simulink model "Demo_PreScanCarSim3D_cs"  (Simulink 7.6)
settings: Solver=ode5  SolverMode=SingleTasking  StartTime=0.0  StopTime=68  FixedStep=1/400  RelTol=1e-3
PreLoadFcn:
  | check_NUTS_defined;
  | 
  | assignin('base',['model_closed_' bdroot],false);
InitFcn:
  | PreScanExperimentInitFcn(bdroot)
StopFcn:
  | PreScanExperimentStopFcn(bdroot)
undefined symbols (not defined in the file or in its folder): DiscIntNeverNeededParam, warningInitialVelocity, x0, x_ini_VRML, y_ini_VRML, z_ini_VRML
libraries: PreScanSimulinkLibrary x13, simulink_extras x5, PreScanUsefulBlocks x5, simulink x3, Solver_SF x1
(part 2 of 10)

== system Demo_PreScanCarSim3D_cs/GetSensors ==
  dummy : Inport
  GetSensors : M-S-Function  FunctionName=GetSensorsBlock  Parameters=TimeStep NrOfSensors
  tag scope: SimCoreSensors=global
  wires:
  GetSensors/1 -> [SimCoreSensors]
  dummy/1 -> GetSensors/1

== system Demo_PreScanCarSim3D_cs/HighwayOverhang_1 ==
  note: Resources
      |
      | 3: InformationSign\MatrixSign_Empty.png: MatrixSign Empty
      | 4: InformationSign\MatrixSign_End.png: MatrixSign End
      | 5: InformationSign\MatrixSign_GreenArrow.png: MatrixSign GreenArrow
      | 6: InformationSign\MatrixSign_RedCross.png: MatrixSign RedCross
      | 7: InformationSign\MatrixSign_Speed_50.png: MatrixSign Speed 50
      | 8: InformationSign\MatrixSign_Speed_70.png: MatrixSign Speed 70
      | 9: InformationSign\MatrixSign_Speed_90.png: MatrixSign Speed 90
      | 10: InformationSign\MatrixSign_Speed_120.png: MatrixSign Speed 120
      | 11: InformationSign\MatrixSign_Speed_130.png: MatrixSign Speed 130
      | 12: InformationSign\information.png: information
      | 13: InformationSign\TASS-international-logo.bmp: TASS-international-logo
  note: Resources
  Ground_{1..8} (8 alike) : Ground
  VISUMatrixSignLights_Mux : Subsystem  Tag=MuxMatrixSignLights
      settings: DeleteFcn=PreScanBlockDeleteFcn;
      mask Type: PreScan Mux Block:
  VISUMatrixSign_Mux : Subsystem  Tag=MuxMatrixSign
      settings: DeleteFcn=PreScanBlockDeleteFcn;
      mask Type: PreScan Mux Block:
  VISUMatrixSign_HighwayOverhang_1 : Outport  Tag=VisuMatrixSignOutport  SampleTime=20/400
  VISUMatrixSignLights_HighwayOverhang_1 : Outport  Tag=VisuMatrixSignLightsOutport  Port=2  SampleTime=20/400
  wires:
  Ground_8/1 -> VISUMatrixSign_Mux/4(MatrixSign_4)
  Ground_7/1 -> VISUMatrixSign_Mux/3(MatrixSign_3)
  Ground_6/1 -> VISUMatrixSign_Mux/2(MatrixSign_2)
  Ground_5/1 -> VISUMatrixSign_Mux/1(MatrixSign_1)
  Ground_4/1 -> VISUMatrixSignLights_Mux/4(MatrixSign_4)
  Ground_3/1 -> VISUMatrixSignLights_Mux/3(MatrixSign_3)
  Ground_2/1 -> VISUMatrixSignLights_Mux/2(MatrixSign_2)
  Ground_1/1 -> VISUMatrixSignLights_Mux/1(MatrixSign_1)
  VISUMatrixSignLights_Mux/1(MatrixSignLights) -> VISUMatrixSignLights_HighwayOverhang_1/1
  VISUMatrixSign_Mux/1(MatrixSigns) -> VISUMatrixSign_HighwayOverhang_1/1

== system Demo_PreScanCarSim3D_cs/HighwayOverhang_2 ==
  note: Resources
      |
      | 3: InformationSign\MatrixSign_Empty.png: MatrixSign Empty
      | 4: InformationSign\MatrixSign_End.png: MatrixSign End
      | 5: InformationSign\MatrixSign_GreenArrow.png: MatrixSign GreenArrow
      | 6: InformationSign\MatrixSign_RedCross.png: MatrixSign RedCross
      | 7: InformationSign\MatrixSign_Speed_50.png: MatrixSign Speed 50
      | 8: InformationSign\MatrixSign_Speed_70.png: MatrixSign Speed 70
      | 9: InformationSign\MatrixSign_Speed_90.png: MatrixSign Speed 90
      | 10: InformationSign\MatrixSign_Speed_120.png: MatrixSign Speed 120
      | 11: InformationSign\MatrixSign_Speed_130.png: MatrixSign Speed 130
      | 12: InformationSign\information.png: information
      | 13: InformationSign\TASS-international-logo.bmp: TASS-international-logo
  note: Resources
  Ground_{1..6} (6 alike) : Ground
  VISUMatrixSignLights_Mux : Subsystem  Tag=MuxMatrixSignLights
      settings: DeleteFcn=PreScanBlockDeleteFcn;
      mask Type: PreScan Mux Block:
  VISUMatrixSign_Mux : Subsystem  Tag=MuxMatrixSign
      settings: DeleteFcn=PreScanBlockDeleteFcn;
      mask Type: PreScan Mux Block:
  VISUMatrixSign_HighwayOverhang_2 : Outport  Tag=VisuMatrixSignOutport  SampleTime=20/400
  VISUMatrixSignLights_HighwayOverhang_2 : Outport  Tag=VisuMatrixSignLightsOutport  Port=2  SampleTime=20/400
  wires:
  Ground_6/1 -> VISUMatrixSign_Mux/3(MatrixSign_7)
  Ground_5/1 -> VISUMatrixSign_Mux/2(MatrixSign_6)
  Ground_4/1 -> VISUMatrixSign_Mux/1(MatrixSign_5)
  Ground_3/1 -> VISUMatrixSignLights_Mux/3(MatrixSign_7)
  Ground_2/1 -> VISUMatrixSignLights_Mux/2(MatrixSign_6)
  Ground_1/1 -> VISUMatrixSignLights_Mux/1(MatrixSign_5)
  VISUMatrixSignLights_Mux/1(MatrixSignLights) -> VISUMatrixSignLights_HighwayOverhang_2/1
  VISUMatrixSign_Mux/1(MatrixSigns) -> VISUMatrixSign_HighwayOverhang_2/1

== system Demo_PreScanCarSim3D_cs/HighwayOverhang_3 ==
  note: Resources
      |
      | 3: InformationSign\MatrixSign_Empty.png: MatrixSign Empty
      | 4: InformationSign\MatrixSign_End.png: MatrixSign End
      | 5: InformationSign\MatrixSign_GreenArrow.png: MatrixSign GreenArrow
      | 6: InformationSign\MatrixSign_RedCross.png: MatrixSign RedCross
      | 7: InformationSign\MatrixSign_Speed_50.png: MatrixSign Speed 50
      | 8: InformationSign\MatrixSign_Speed_70.png: MatrixSign Speed 70
      | 9: InformationSign\MatrixSign_Speed_90.png: MatrixSign Speed 90
      | 10: InformationSign\MatrixSign_Speed_120.png: MatrixSign Speed 120
      | 11: InformationSign\MatrixSign_Speed_130.png: MatrixSign Speed 130
      | 12: InformationSign\information.png: information
      | 13: InformationSign\TASS-international-logo.bmp: TASS-international-logo
  note: Resources
  Ground_{1..6} (6 alike) : Ground
  VISUMatrixSignLights_Mux : Subsystem  Tag=MuxMatrixSignLights
      settings: DeleteFcn=PreScanBlockDeleteFcn;
      mask Type: PreScan Mux Block:
  VISUMatrixSign_Mux : Subsystem  Tag=MuxMatrixSign
      settings: DeleteFcn=PreScanBlockDeleteFcn;
      mask Type: PreScan Mux Block:
  VISUMatrixSign_HighwayOverhang_3 : Outport  Tag=VisuMatrixSignOutport  SampleTime=20/400
  VISUMatrixSignLights_HighwayOverhang_3 : Outport  Tag=VisuMatrixSignLightsOutport  Port=2  SampleTime=20/400
  wires:
  Ground_6/1 -> VISUMatrixSign_Mux/3(MatrixSign_12)
  Ground_5/1 -> VISUMatrixSign_Mux/2(MatrixSign_11)
  Ground_4/1 -> VISUMatrixSign_Mux/1(MatrixSign_10)
  Ground_3/1 -> VISUMatrixSignLights_Mux/3(MatrixSign_12)
  Ground_2/1 -> VISUMatrixSignLights_Mux/2(MatrixSign_11)
  Ground_1/1 -> VISUMatrixSignLights_Mux/1(MatrixSign_10)
  VISUMatrixSignLights_Mux/1(MatrixSignLights) -> VISUMatrixSignLights_HighwayOverhang_3/1
  VISUMatrixSign_Mux/1(MatrixSigns) -> VISUMatrixSign_HighwayOverhang_3/1

== system Demo_PreScanCarSim3D_cs/HighwayOverhang_5 ==
  note: Resources
      |
      | 3: InformationSign\MatrixSign_Empty.png: MatrixSign Empty
      | 4: InformationSign\MatrixSign_End.png: MatrixSign End
      | 5: InformationSign\MatrixSign_GreenArrow.png: MatrixSign GreenArrow
      | 6: InformationSign\MatrixSign_RedCross.png: MatrixSign RedCross
      | 7: InformationSign\MatrixSign_Speed_50.png: MatrixSign Speed 50
      | 8: InformationSign\MatrixSign_Speed_70.png: MatrixSign Speed 70
      | 9: InformationSign\MatrixSign_Speed_90.png: MatrixSign Speed 90
      | 10: InformationSign\MatrixSign_Speed_120.png: MatrixSign Speed 120
      | 11: InformationSign\MatrixSign_Speed_130.png: MatrixSign Speed 130
      | 12: InformationSign\information.png: information
      | 13: InformationSign\TASS-international-logo.bmp: TASS-international-logo
  note: Resources
  Ground_{1..6} (6 alike) : Ground
  VISUMatrixSignLights_Mux : Subsystem  Tag=MuxMatrixSignLights
      settings: DeleteFcn=PreScanBlockDeleteFcn;
      mask Type: PreScan Mux Block:
  VISUMatrixSign_Mux : Subsystem  Tag=MuxMatrixSign
      settings: DeleteFcn=PreScanBlockDeleteFcn;
      mask Type: PreScan Mux Block:
  VISUMatrixSign_HighwayOverhang_5 : Outport  Tag=VisuMatrixSignOutport  SampleTime=20/400
  VISUMatrixSignLights_HighwayOverhang_5 : Outport  Tag=VisuMatrixSignLightsOutport  Port=2  SampleTime=20/400
  wires:
  Ground_6/1 -> VISUMatrixSign_Mux/3(MatrixSign_20)
  Ground_5/1 -> VISUMatrixSign_Mux/2(MatrixSign_19)
  Ground_4/1 -> VISUMatrixSign_Mux/1(MatrixSign_18)
  Ground_3/1 -> VISUMatrixSignLights_Mux/3(MatrixSign_20)
  Ground_2/1 -> VISUMatrixSignLights_Mux/2(MatrixSign_19)
  Ground_1/1 -> VISUMatrixSignLights_Mux/1(MatrixSign_18)
  VISUMatrixSignLights_Mux/1(MatrixSignLights) -> VISUMatrixSignLights_HighwayOverhang_5/1
  VISUMatrixSign_Mux/1(MatrixSigns) -> VISUMatrixSign_HighwayOverhang_5/1

== system Demo_PreScanCarSim3D_cs/Lightpost_1 ==

== system Demo_PreScanCarSim3D_cs/Lightpost_10 ==

== system Demo_PreScanCarSim3D_cs/Lightpost_11 ==

== system Demo_PreScanCarSim3D_cs/Lightpost_12 ==

== system Demo_PreScanCarSim3D_cs/Lightpost_13 ==

== system Demo_PreScanCarSim3D_cs/Lightpost_14 ==

== system Demo_PreScanCarSim3D_cs/Lightpost_15 ==

== system Demo_PreScanCarSim3D_cs/Lightpost_16 ==

== system Demo_PreScanCarSim3D_cs/Lightpost_17 ==

== system Demo_PreScanCarSim3D_cs/Lightpost_18 ==

== system Demo_PreScanCarSim3D_cs/Lightpost_19 ==

== system Demo_PreScanCarSim3D_cs/Lightpost_2 ==

== system Demo_PreScanCarSim3D_cs/Lightpost_20 ==

== system Demo_PreScanCarSim3D_cs/Lightpost_21 ==

== system Demo_PreScanCarSim3D_cs/Lightpost_22 ==

== system Demo_PreScanCarSim3D_cs/Lightpost_23 ==

== system Demo_PreScanCarSim3D_cs/Lightpost_24 ==

== system Demo_PreScanCarSim3D_cs/Lightpost_25 ==

== system Demo_PreScanCarSim3D_cs/Lightpost_26 ==

== system Demo_PreScanCarSim3D_cs/Lightpost_27 ==

== system Demo_PreScanCarSim3D_cs/Lightpost_28 ==

== system Demo_PreScanCarSim3D_cs/Lightpost_29 ==

== system Demo_PreScanCarSim3D_cs/Lightpost_30 ==

== system Demo_PreScanCarSim3D_cs/Lightpost_31 ==

== system Demo_PreScanCarSim3D_cs/Lightpost_32 ==

== system Demo_PreScanCarSim3D_cs/Lightpost_33 ==

== system Demo_PreScanCarSim3D_cs/Lightpost_34 ==

== system Demo_PreScanCarSim3D_cs/Lightpost_35 ==

== system Demo_PreScanCarSim3D_cs/Lightpost_36 ==

== system Demo_PreScanCarSim3D_cs/Lightpost_7 ==

== system Demo_PreScanCarSim3D_cs/Lightpost_8 ==

== system Demo_PreScanCarSim3D_cs/Lightpost_9 ==

== system Demo_PreScanCarSim3D_cs/SELF_Audi_A8_1 ==
  Selector : Selector  IndexMode=Zero-based  IndexOptions=Starting index (dialog)  Indices=PortIndex  OutputSizes=PortWidth(1)
  U : Outport
  wires:
  Selector/1 -> U/1
  [SimCoreSensors] -> Selector/1

== system Demo_PreScanCarSim3D_cs/SELF_Box_1 ==
  Selector : Selector  IndexMode=Zero-based  IndexOptions=Starting index (dialog)  Indices=PortIndex  OutputSizes=PortWidth(1)
  U : Outport
  wires:
  Selector/1 -> U/1
  [SimCoreSensors] -> Selector/1

== system Demo_PreScanCarSim3D_cs/SELF_Box_2 ==
  Selector : Selector  IndexMode=Zero-based  IndexOptions=Starting index (dialog)  Indices=PortIndex  OutputSizes=PortWidth(1)
  U : Outport
  wires:
  Selector/1 -> U/1
  [SimCoreSensors] -> Selector/1

== system Demo_PreScanCarSim3D_cs/SELF_Box_3 ==
  Selector : Selector  IndexMode=Zero-based  IndexOptions=Starting index (dialog)  Indices=PortIndex  OutputSizes=PortWidth(1)
  U : Outport
  wires:
  Selector/1 -> U/1
  [SimCoreSensors] -> Selector/1

== system Demo_PreScanCarSim3D_cs/SELF_Box_4 ==
  Selector : Selector  IndexMode=Zero-based  IndexOptions=Starting index (dialog)  Indices=PortIndex  OutputSizes=PortWidth(1)
  U : Outport
  wires:
  Selector/1 -> U/1
  [SimCoreSensors] -> Selector/1

== system Demo_PreScanCarSim3D_cs/STATE_Audi_A8_1 ==
  State : Inport  SampleTime=TimeStep
  Acceleration : Subsystem  mask(ToSensorWorld){PortName=Acceleration_Audi_A8_1, PortIndex=66, PortWidth=3, TimeStep=20/400}
      mask prompts: PortName "Port Name [-]"; PortIndex "Index [-]"; PortWidth "Port Dimensions [-]"; TimeStep "Upload Period [s]"
      mask help: Sends signal(s) from Simulink to the Sensor World
      mask Help:
      | Sends signal(s) from Simulink to the Sensor World.
      | 
      | - Port Name [-]: specifies the name of the output terminal of the Simulink block.
      | - Index [-]: specifies the start position in the output vector sent to the Sensor World
      | - Port dimensions [-]: specifies the width (number of scalars) of the output port
      | - Upload period [s]: specifies the upload period (in seconds) of the port.
      mask Display: port_label('input', 1, PortName)
  Demux : Demux  Outputs=5
  Position : Subsystem  mask(ToSensorWorld){PortName=Position_Audi_A8_1, PortIndex=60, PortWidth=3, TimeStep=20/400}
      mask prompts: PortName "Port Name [-]"; PortIndex "Index [-]"; PortWidth "Port Dimensions [-]"; TimeStep "Upload Period [s]"
      mask help: Sends signal(s) from Simulink to the Sensor World
      mask Help:
      | Sends signal(s) from Simulink to the Sensor World.
      | 
      | - Port Name [-]: specifies the name of the output terminal of the Simulink block.
      | - Index [-]: specifies the start position in the output vector sent to the Sensor World
      | - Port dimensions [-]: specifies the width (number of scalars) of the output port
      | - Upload period [s]: specifies the upload period (in seconds) of the port.
      mask Display: port_label('input', 1, PortName)
  RPY : Subsystem  mask(ToSensorWorld){PortName=RPY_Audi_A8_1, PortIndex=69, PortWidth=3, TimeStep=20/400}
      mask prompts: PortName "Port Name [-]"; PortIndex "Index [-]"; PortWidth "Port Dimensions [-]"; TimeStep "Upload Period [s]"
      mask help: Sends signal(s) from Simulink to the Sensor World
      mask Help:
      | Sends signal(s) from Simulink to the Sensor World.
      | 
      | - Port Name [-]: specifies the name of the output terminal of the Simulink block.
      | - Index [-]: specifies the start position in the output vector sent to the Sensor World
      | - Port dimensions [-]: specifies the width (number of scalars) of the output port
      | - Upload period [s]: specifies the upload period (in seconds) of the port.
      mask Display: port_label('input', 1, PortName)
  Velocity : Subsystem  mask(ToSensorWorld){PortName=Velocity_Audi_A8_1, PortIndex=63, PortWidth=3, TimeStep=20/400}
      mask prompts: PortName "Port Name [-]"; PortIndex "Index [-]"; PortWidth "Port Dimensions [-]"; TimeStep "Upload Period [s]"
      mask help: Sends signal(s) from Simulink to the Sensor World
      mask Help:
      | Sends signal(s) from Simulink to the Sensor World.
      | 
      | - Port Name [-]: specifies the name of the output terminal of the Simulink block.
      | - Index [-]: specifies the start position in the output vector sent to the Sensor World
      | - Port dimensions [-]: specifies the width (number of scalars) of the output port
      | - Upload period [s]: specifies the upload period (in seconds) of the port.
      mask Display: port_label('input', 1, PortName)
  iniBODYAngles wrtVEH [rad] : Constant  Value=[Roll0 Pitch0 0]  SampleTime=TimeStep
  iniVEHAngles wrtGLOB [rad] : Constant  Value=[0 0 Yaw0]  SampleTime=TimeStep
  iniVEHposition wrtGLOB [m] : Constant  Value=[x0 y0 z0]  SampleTime=TimeStep
  state2FullState : PreScanSimulinkLibrary/state2FullState  SystemSampleTime=-1
  velRPY : Subsystem  mask(ToSensorWorld){PortName=velRPY_Audi_A8_1, PortIndex=72, PortWidth=3, TimeStep=20/400}
      mask prompts: PortName "Port Name [-]"; PortIndex "Index [-]"; PortWidth "Port Dimensions [-]"; TimeStep "Upload Period [s]"
      mask help: Sends signal(s) from Simulink to the Sensor World
      mask Help:
      | Sends signal(s) from Simulink to the Sensor World.
      | 
      | - Port Name [-]: specifies the name of the output terminal of the Simulink block.
      | - Index [-]: specifies the start position in the output vector sent to the Sensor World
      | - Port dimensions [-]: specifies the width (number of scalars) of the output port
      | - Upload period [s]: specifies the upload period (in seconds) of the port.
      mask Display: port_label('input', 1, PortName)
  wires:
  Demux/5 -> velRPY/1(Y)
  Demux/4 -> RPY/1(Y)
  Demux/3 -> Acceleration/1(Y)
  Demux/2 -> Velocity/1(Y)
  Demux/1 -> Position/1(Y)
  State/1 -> state2FullState/1
  state2FullState/1 -> Demux/1
  iniVEHposition wrtGLOB [m]/1 -> state2FullState/2
  iniBODYAngles wrtVEH [rad]/1 -> state2FullState/3
  iniVEHAngles wrtGLOB [rad]/1 -> state2FullState/4

== system Demo_PreScanCarSim3D_cs/STATE_Box_1 ==
  State : Inport  SampleTime=TimeStep
  Acceleration : Subsystem  mask(ToSensorWorld){PortName=Acceleration_Box_1, PortIndex=6, PortWidth=3, TimeStep=20/400}
      mask prompts: PortName "Port Name [-]"; PortIndex "Index [-]"; PortWidth "Port Dimensions [-]"; TimeStep "Upload Period [s]"
      mask help: Sends signal(s) from Simulink to the Sensor World
      mask Help:
      | Sends signal(s) from Simulink to the Sensor World.
      | 
      | - Port Name [-]: specifies the name of the output terminal of the Simulink block.
      | - Index [-]: specifies the start position in the output vector sent to the Sensor World
      | - Port dimensions [-]: specifies the width (number of scalars) of the output port
      | - Upload period [s]: specifies the upload period (in seconds) of the port.
      mask Display: port_label('input', 1, PortName)
  Demux : Demux  Outputs=5
  Position : Subsystem  mask(ToSensorWorld){PortName=Position_Box_1, PortIndex=0, PortWidth=3, TimeStep=20/400}
      mask prompts: PortName "Port Name [-]"; PortIndex "Index [-]"; PortWidth "Port Dimensions [-]"; TimeStep "Upload Period [s]"
      mask help: Sends signal(s) from Simulink to the Sensor World
      mask Help:
      | Sends signal(s) from Simulink to the Sensor World.
      | 
      | - Port Name [-]: specifies the name of the output terminal of the Simulink block.
      | - Index [-]: specifies the start position in the output vector sent to the Sensor World
      | - Port dimensions [-]: specifies the width (number of scalars) of the output port
      | - Upload period [s]: specifies the upload period (in seconds) of the port.
      mask Display: port_label('input', 1, PortName)
  RPY : Subsystem  mask(ToSensorWorld){PortName=RPY_Box_1, PortIndex=9, PortWidth=3, TimeStep=20/400}
      mask prompts: PortName "Port Name [-]"; PortIndex "Index [-]"; PortWidth "Port Dimensions [-]"; TimeStep "Upload Period [s]"
      mask help: Sends signal(s) from Simulink to the Sensor World
      mask Help:
      | Sends signal(s) from Simulink to the Sensor World.
      | 
      | - Port Name [-]: specifies the name of the output terminal of the Simulink block.
      | - Index [-]: specifies the start position in the output vector sent to the Sensor World
      | - Port dimensions [-]: specifies the width (number of scalars) of the output port
      | - Upload period [s]: specifies the upload period (in seconds) of the port.
      mask Display: port_label('input', 1, PortName)
  Velocity : Subsystem  mask(ToSensorWorld){PortName=Velocity_Box_1, PortIndex=3, PortWidth=3, TimeStep=20/400}
      mask prompts: PortName "Port Name [-]"; PortIndex "Index [-]"; PortWidth "Port Dimensions [-]"; TimeStep "Upload Period [s]"
      mask help: Sends signal(s) from Simulink to the Sensor World
      mask Help:
      | Sends signal(s) from Simulink to the Sensor World.
      | 
      | - Port Name [-]: specifies the name of the output terminal of the Simulink block.
      | - Index [-]: specifies the start position in the output vector sent to the Sensor World
      | - Port dimensions [-]: specifies the width (number of scalars) of the output port
      | - Upload period [s]: specifies the upload period (in seconds) of the port.
      mask Display: port_label('input', 1, PortName)
  iniBODYAngles wrtVEH [rad] : Constant  Value=[Roll0 Pitch0 0]  SampleTime=TimeStep
  iniVEHAngles wrtGLOB [rad] : Constant  Value=[0 0 Yaw0]  SampleTime=TimeStep
  iniVEHposition wrtGLOB [m] : Constant  Value=[x0 y0 z0]  SampleTime=TimeStep
  state2FullState : PreScanSimulinkLibrary/state2FullState  SystemSampleTime=-1
  velRPY : Subsystem  mask(ToSensorWorld){PortName=velRPY_Box_1, PortIndex=12, PortWidth=3, TimeStep=20/400}
      mask prompts: PortName "Port Name [-]"; PortIndex "Index [-]"; PortWidth "Port Dimensions [-]"; TimeStep "Upload Period [s]"
      mask help: Sends signal(s) from Simulink to the Sensor World
      mask Help:
      | Sends signal(s) from Simulink to the Sensor World.
      | 
      | - Port Name [-]: specifies the name of the output terminal of the Simulink block.
      | - Index [-]: specifies the start position in the output vector sent to the Sensor World
      | - Port dimensions [-]: specifies the width (number of scalars) of the output port
      | - Upload period [s]: specifies the upload period (in seconds) of the port.
      mask Display: port_label('input', 1, PortName)
  wires:
  Demux/5 -> velRPY/1(Y)
  Demux/4 -> RPY/1(Y)
  Demux/3 -> Acceleration/1(Y)
  Demux/2 -> Velocity/1(Y)
  Demux/1 -> Position/1(Y)
  State/1 -> state2FullState/1
  state2FullState/1 -> Demux/1
  iniVEHposition wrtGLOB [m]/1 -> state2FullState/2
  iniBODYAngles wrtVEH [rad]/1 -> state2FullState/3
  iniVEHAngles wrtGLOB [rad]/1 -> state2FullState/4

== system Demo_PreScanCarSim3D_cs/STATE_Box_2 ==
  State : Inport  SampleTime=TimeStep
  Acceleration : Subsystem  mask(ToSensorWorld){PortName=Acceleration_Box_2, PortIndex=21, PortWidth=3, TimeStep=20/400}
      mask prompts: PortName "Port Name [-]"; PortIndex "Index [-]"; PortWidth "Port Dimensions [-]"; TimeStep "Upload Period [s]"
      mask help: Sends signal(s) from Simulink to the Sensor World
      mask Help:
      | Sends signal(s) from Simulink to the Sensor World.
      | 
      | - Port Name [-]: specifies the name of the output terminal of the Simulink block.
      | - Index [-]: specifies the start position in the output vector sent to the Sensor World
      | - Port dimensions [-]: specifies the width (number of scalars) of the output port
      | - Upload period [s]: specifies the upload period (in seconds) of the port.
      mask Display: port_label('input', 1, PortName)
  Demux : Demux  Outputs=5
  Position : Subsystem  mask(ToSensorWorld){PortName=Position_Box_2, PortIndex=15, PortWidth=3, TimeStep=20/400}
      mask prompts: PortName "Port Name [-]"; PortIndex "Index [-]"; PortWidth "Port Dimensions [-]"; TimeStep "Upload Period [s]"
      mask help: Sends signal(s) from Simulink to the Sensor World
      mask Help:
      | Sends signal(s) from Simulink to the Sensor World.
      | 
      | - Port Name [-]: specifies the name of the output terminal of the Simulink block.
      | - Index [-]: specifies the start position in the output vector sent to the Sensor World
      | - Port dimensions [-]: specifies the width (number of scalars) of the output port
      | - Upload period [s]: specifies the upload period (in seconds) of the port.
      mask Display: port_label('input', 1, PortName)
  RPY : Subsystem  mask(ToSensorWorld){PortName=RPY_Box_2, PortIndex=24, PortWidth=3, TimeStep=20/400}
      mask prompts: PortName "Port Name [-]"; PortIndex "Index [-]"; PortWidth "Port Dimensions [-]"; TimeStep "Upload Period [s]"
      mask help: Sends signal(s) from Simulink to the Sensor World
      mask Help:
      | Sends signal(s) from Simulink to the Sensor World.
      | 
      | - Port Name [-]: specifies the name of the output terminal of the Simulink block.
      | - Index [-]: specifies the start position in the output vector sent to the Sensor World
      | - Port dimensions [-]: specifies the width (number of scalars) of the output port
      | - Upload period [s]: specifies the upload period (in seconds) of the port.
      mask Display: port_label('input', 1, PortName)
  Velocity : Subsystem  mask(ToSensorWorld){PortName=Velocity_Box_2, PortIndex=18, PortWidth=3, TimeStep=20/400}
      mask prompts: PortName "Port Name [-]"; PortIndex "Index [-]"; PortWidth "Port Dimensions [-]"; TimeStep "Upload Period [s]"
      mask help: Sends signal(s) from Simulink to the Sensor World
      mask Help:
      | Sends signal(s) from Simulink to the Sensor World.
      | 
      | - Port Name [-]: specifies the name of the output terminal of the Simulink block.
      | - Index [-]: specifies the start position in the output vector sent to the Sensor World
      | - Port dimensions [-]: specifies the width (number of scalars) of the output port
      | - Upload period [s]: specifies the upload period (in seconds) of the port.
      mask Display: port_label('input', 1, PortName)
  iniBODYAngles wrtVEH [rad] : Constant  Value=[Roll0 Pitch0 0]  SampleTime=TimeStep
  iniVEHAngles wrtGLOB [rad] : Constant  Value=[0 0 Yaw0]  SampleTime=TimeStep
  iniVEHposition wrtGLOB [m] : Constant  Value=[x0 y0 z0]  SampleTime=TimeStep
  state2FullState : PreScanSimulinkLibrary/state2FullState  SystemSampleTime=-1
  velRPY : Subsystem  mask(ToSensorWorld){PortName=velRPY_Box_2, PortIndex=27, PortWidth=3, TimeStep=20/400}
      mask prompts: PortName "Port Name [-]"; PortIndex "Index [-]"; PortWidth "Port Dimensions [-]"; TimeStep "Upload Period [s]"
      mask help: Sends signal(s) from Simulink to the Sensor World
      mask Help:
      | Sends signal(s) from Simulink to the Sensor World.
      | 
      | - Port Name [-]: specifies the name of the output terminal of the Simulink block.
      | - Index [-]: specifies the start position in the output vector sent to the Sensor World
      | - Port dimensions [-]: specifies the width (number of scalars) of the output port
      | - Upload period [s]: specifies the upload period (in seconds) of the port.
      mask Display: port_label('input', 1, PortName)
  wires:
  Demux/5 -> velRPY/1(Y)
  Demux/4 -> RPY/1(Y)
  Demux/3 -> Acceleration/1(Y)
  Demux/2 -> Velocity/1(Y)
  Demux/1 -> Position/1(Y)
  State/1 -> state2FullState/1
  state2FullState/1 -> Demux/1
  iniVEHposition wrtGLOB [m]/1 -> state2FullState/2
  iniBODYAngles wrtVEH [rad]/1 -> state2FullState/3
  iniVEHAngles wrtGLOB [rad]/1 -> state2FullState/4

== system Demo_PreScanCarSim3D_cs/STATE_Box_3 ==
  State : Inport  SampleTime=TimeStep
  Acceleration : Subsystem  mask(ToSensorWorld){PortName=Acceleration_Box_3, PortIndex=36, PortWidth=3, TimeStep=20/400}
      mask prompts: PortName "Port Name [-]"; PortIndex "Index [-]"; PortWidth "Port Dimensions [-]"; TimeStep "Upload Period [s]"
      mask help: Sends signal(s) from Simulink to the Sensor World
      mask Help:
      | Sends signal(s) from Simulink to the Sensor World.
      | 
      | - Port Name [-]: specifies the name of the output terminal of the Simulink block.
      | - Index [-]: specifies the start position in the output vector sent to the Sensor World
      | - Port dimensions [-]: specifies the width (number of scalars) of the output port
      | - Upload period [s]: specifies the upload period (in seconds) of the port.
      mask Display: port_label('input', 1, PortName)
  Demux : Demux  Outputs=5
  Position : Subsystem  mask(ToSensorWorld){PortName=Position_Box_3, PortIndex=30, PortWidth=3, TimeStep=20/400}
      mask prompts: PortName "Port Name [-]"; PortIndex "Index [-]"; PortWidth "Port Dimensions [-]"; TimeStep "Upload Period [s]"
      mask help: Sends signal(s) from Simulink to the Sensor World
      mask Help:
      | Sends signal(s) from Simulink to the Sensor World.
      | 
      | - Port Name [-]: specifies the name of the output terminal of the Simulink block.
      | - Index [-]: specifies the start position in the output vector sent to the Sensor World
      | - Port dimensions [-]: specifies the width (number of scalars) of the output port
      | - Upload period [s]: specifies the upload period (in seconds) of the port.
      mask Display: port_label('input', 1, PortName)
  RPY : Subsystem  mask(ToSensorWorld){PortName=RPY_Box_3, PortIndex=39, PortWidth=3, TimeStep=20/400}
      mask prompts: PortName "Port Name [-]"; PortIndex "Index [-]"; PortWidth "Port Dimensions [-]"; TimeStep "Upload Period [s]"
      mask help: Sends signal(s) from Simulink to the Sensor World
      mask Help:
      | Sends signal(s) from Simulink to the Sensor World.
      | 
      | - Port Name [-]: specifies the name of the output terminal of the Simulink block.
      | - Index [-]: specifies the start position in the output vector sent to the Sensor World
      | - Port dimensions [-]: specifies the width (number of scalars) of the output port
      | - Upload period [s]: specifies the upload period (in seconds) of the port.
      mask Display: port_label('input', 1, PortName)
  Velocity : Subsystem  mask(ToSensorWorld){PortName=Velocity_Box_3, PortIndex=33, PortWidth=3, TimeStep=20/400}
      mask prompts: PortName "Port Name [-]"; PortIndex "Index [-]"; PortWidth "Port Dimensions [-]"; TimeStep "Upload Period [s]"
      mask help: Sends signal(s) from Simulink to the Sensor World
      mask Help:
      | Sends signal(s) from Simulink to the Sensor World.
      | 
      | - Port Name [-]: specifies the name of the output terminal of the Simulink block.
      | - Index [-]: specifies the start position in the output vector sent to the Sensor World
      | - Port dimensions [-]: specifies the width (number of scalars) of the output port
      | - Upload period [s]: specifies the upload period (in seconds) of the port.
      mask Display: port_label('input', 1, PortName)
  iniBODYAngles wrtVEH [rad] : Constant  Value=[Roll0 Pitch0 0]  SampleTime=TimeStep
  iniVEHAngles wrtGLOB [rad] : Constant  Value=[0 0 Yaw0]  SampleTime=TimeStep
  iniVEHposition wrtGLOB [m] : Constant  Value=[x0 y0 z0]  SampleTime=TimeStep
  state2FullState : PreScanSimulinkLibrary/state2FullState  SystemSampleTime=-1
  velRPY : Subsystem  mask(ToSensorWorld){PortName=velRPY_Box_3, PortIndex=42, PortWidth=3, TimeStep=20/400}
      mask prompts: PortName "Port Name [-]"; PortIndex "Index [-]"; PortWidth "Port Dimensions [-]"; TimeStep "Upload Period [s]"
      mask help: Sends signal(s) from Simulink to the Sensor World
      mask Help:
      | Sends signal(s) from Simulink to the Sensor World.
      | 
      | - Port Name [-]: specifies the name of the output terminal of the Simulink block.
      | - Index [-]: specifies the start position in the output vector sent to the Sensor World
      | - Port dimensions [-]: specifies the width (number of scalars) of the output port
      | - Upload period [s]: specifies the upload period (in seconds) of the port.
      mask Display: port_label('input', 1, PortName)
  wires:
  Demux/5 -> velRPY/1(Y)
  Demux/4 -> RPY/1(Y)
  Demux/3 -> Acceleration/1(Y)
  Demux/2 -> Velocity/1(Y)
  Demux/1 -> Position/1(Y)
  State/1 -> state2FullState/1
  state2FullState/1 -> Demux/1
  iniVEHposition wrtGLOB [m]/1 -> state2FullState/2
  iniBODYAngles wrtVEH [rad]/1 -> state2FullState/3
  iniVEHAngles wrtGLOB [rad]/1 -> state2FullState/4

== system Demo_PreScanCarSim3D_cs/STATE_Box_4 ==
  State : Inport  SampleTime=TimeStep
  Acceleration : Subsystem  mask(ToSensorWorld){PortName=Acceleration_Box_4, PortIndex=51, PortWidth=3, TimeStep=20/400}
      mask prompts: PortName "Port Name [-]"; PortIndex "Index [-]"; PortWidth "Port Dimensions [-]"; TimeStep "Upload Period [s]"
      mask help: Sends signal(s) from Simulink to the Sensor World
      mask Help:
      | Sends signal(s) from Simulink to the Sensor World.
      | 
      | - Port Name [-]: specifies the name of the output terminal of the Simulink block.
      | - Index [-]: specifies the start position in the output vector sent to the Sensor World
      | - Port dimensions [-]: specifies the width (number of scalars) of the output port
      | - Upload period [s]: specifies the upload period (in seconds) of the port.
      mask Display: port_label('input', 1, PortName)
  Demux : Demux  Outputs=5
  Position : Subsystem  mask(ToSensorWorld){PortName=Position_Box_4, PortIndex=45, PortWidth=3, TimeStep=20/400}
      mask prompts: PortName "Port Name [-]"; PortIndex "Index [-]"; PortWidth "Port Dimensions [-]"; TimeStep "Upload Period [s]"
      mask help: Sends signal(s) from Simulink to the Sensor World
      mask Help:
      | Sends signal(s) from Simulink to the Sensor World.
      | 
      | - Port Name [-]: specifies the name of the output terminal of the Simulink block.
      | - Index [-]: specifies the start position in the output vector sent to the Sensor World
      | - Port dimensions [-]: specifies the width (number of scalars) of the output port
      | - Upload period [s]: specifies the upload period (in seconds) of the port.
      mask Display: port_label('input', 1, PortName)
  RPY : Subsystem  mask(ToSensorWorld){PortName=RPY_Box_4, PortIndex=54, PortWidth=3, TimeStep=20/400}
      mask prompts: PortName "Port Name [-]"; PortIndex "Index [-]"; PortWidth "Port Dimensions [-]"; TimeStep "Upload Period [s]"
      mask help: Sends signal(s) from Simulink to the Sensor World
      mask Help:
      | Sends signal(s) from Simulink to the Sensor World.
      | 
      | - Port Name [-]: specifies the name of the output terminal of the Simulink block.
      | - Index [-]: specifies the start position in the output vector sent to the Sensor World
      | - Port dimensions [-]: specifies the width (number of scalars) of the output port
      | - Upload period [s]: specifies the upload period (in seconds) of the port.
      mask Display: port_label('input', 1, PortName)
  Velocity : Subsystem  mask(ToSensorWorld){PortName=Velocity_Box_4, PortIndex=48, PortWidth=3, TimeStep=20/400}
      mask prompts: PortName "Port Name [-]"; PortIndex "Index [-]"; PortWidth "Port Dimensions [-]"; TimeStep "Upload Period [s]"
      mask help: Sends signal(s) from Simulink to the Sensor World
      mask Help:
      | Sends signal(s) from Simulink to the Sensor World.
      | 
      | - Port Name [-]: specifies the name of the output terminal of the Simulink block.
      | - Index [-]: specifies the start position in the output vector sent to the Sensor World
      | - Port dimensions [-]: specifies the width (number of scalars) of the output port
      | - Upload period [s]: specifies the upload period (in seconds) of the port.
      mask Display: port_label('input', 1, PortName)
  iniBODYAngles wrtVEH [rad] : Constant  Value=[Roll0 Pitch0 0]  SampleTime=TimeStep
  iniVEHAngles wrtGLOB [rad] : Constant  Value=[0 0 Yaw0]  SampleTime=TimeStep
  iniVEHposition wrtGLOB [m] : Constant  Value=[x0 y0 z0]  SampleTime=TimeStep
  state2FullState : PreScanSimulinkLibrary/state2FullState  SystemSampleTime=-1
  velRPY : Subsystem  mask(ToSensorWorld){PortName=velRPY_Box_4, PortIndex=57, PortWidth=3, TimeStep=20/400}
      mask prompts: PortName "Port Name [-]"; PortIndex "Index [-]"; PortWidth "Port Dimensions [-]"; TimeStep "Upload Period [s]"
      mask help: Sends signal(s) from Simulink to the Sensor World
      mask Help:
      | Sends signal(s) from Simulink to the Sensor World.
      | 
      | - Port Name [-]: specifies the name of the output terminal of the Simulink block.
      | - Index [-]: specifies the start position in the output vector sent to the Sensor World
      | - Port dimensions [-]: specifies the width (number of scalars) of the output port
      | - Upload period [s]: specifies the upload period (in seconds) of the port.
      mask Display: port_label('input', 1, PortName)
  wires:
  Demux/5 -> velRPY/1(Y)
  Demux/4 -> RPY/1(Y)
  Demux/3 -> Acceleration/1(Y)
  Demux/2 -> Velocity/1(Y)
  Demux/1 -> Position/1(Y)
  State/1 -> state2FullState/1
  state2FullState/1 -> Demux/1
  iniVEHposition wrtGLOB [m]/1 -> state2FullState/2
  iniBODYAngles wrtVEH [rad]/1 -> state2FullState/3
  iniVEHAngles wrtGLOB [rad]/1 -> state2FullState/4

== system Demo_PreScanCarSim3D_cs/SetActuators ==
  Bus Creator : BusCreator  Inputs=1
  Data Store Read : DataStoreRead  DataStoreName=SimCoreActuators  SampleTime=TimeStep
  SendActuators : M-S-Function  FunctionName=SendActuatorsBlock  Parameters=TimeStep NrOfActuators
  dummy : Outport
  tag scope: SimCoreInfo=global
  wires:
  Bus Creator/1 -> [SimCoreInfo]  "SimCore"
  SendActuators/2 -> Bus Creator/1  "ComputationTime[s]"
  SendActuators/1 -> dummy/1
  Data Store Read/1 -> SendActuators/1

== system Demo_PreScanCarSim3D_cs/SimCoreInfo ==
  Bus Selector : BusSelector  OutputSignals=ComputationTime[s]
  Time : Scope
      settings: TimeRange=10  YMin=0  YMax=0.5  SaveName=ComputationTime
  wires:
  Bus Selector/1 -> Time/1  "<ComputationTime[s]>"
  [SimCoreInfo] -> Bus Selector/1

== system Demo_PreScanCarSim3D_cs/TrafficLightRoadSideNL_1 ==
  Ground_1 : Ground
  Ground_2 : Ground
  Ground_3 : Ground
  VISUCasingLights_Mux : Subsystem  Tag=MuxCasingLights
      settings: DeleteFcn=PreScanBlockDeleteFcn;
      mask Type: PreScan Mux Block:
  VISUCasingLights_TrafficLightRoadSideNL_1 : Outport  Tag=VisuCasingLightsOutport  SampleTime=20/400
  wires:
  Ground_3/1 -> VISUCasingLights_Mux/3(Green [-])
  Ground_2/1 -> VISUCasingLights_Mux/2(Orange [-])
  Ground_1/1 -> VISUCasingLights_Mux/1(Red [-])
  VISUCasingLights_Mux/1(CasingLights) -> VISUCasingLights_TrafficLightRoadSideNL_1/1

== system Demo_PreScanCarSim3D_cs/TrafficLightRoadSideNL_2 ==
  Ground_1 : Ground
  Ground_2 : Ground
  Ground_3 : Ground
  VISUCasingLights_Mux : Subsystem  Tag=MuxCasingLights
      settings: DeleteFcn=PreScanBlockDeleteFcn;
      mask Type: PreScan Mux Block:
  VISUCasingLights_TrafficLightRoadSideNL_2 : Outport  Tag=VisuCasingLightsOutport  SampleTime=20/400
  wires:
  Ground_3/1 -> VISUCasingLights_Mux/3(Green [-])
  Ground_2/1 -> VISUCasingLights_Mux/2(Orange [-])
  Ground_1/1 -> VISUCasingLights_Mux/1(Red [-])
  VISUCasingLights_Mux/1(CasingLights) -> VISUCasingLights_TrafficLightRoadSideNL_2/1

== system Demo_PreScanCarSim3D_cs/TrafficLightRoadSideNL_3 ==
  Ground_1 : Ground
  Ground_2 : Ground
  Ground_3 : Ground
  VISUCasingLights_Mux : Subsystem  Tag=MuxCasingLights
      settings: DeleteFcn=PreScanBlockDeleteFcn;
      mask Type: PreScan Mux Block:
  VISUCasingLights_TrafficLightRoadSideNL_3 : Outport  Tag=VisuCasingLightsOutport  SampleTime=20/400
  wires:
  Ground_3/1 -> VISUCasingLights_Mux/3(Green [-])
  Ground_2/1 -> VISUCasingLights_Mux/2(Orange [-])
  Ground_1/1 -> VISUCasingLights_Mux/1(Red [-])
  VISUCasingLights_Mux/1(CasingLights) -> VISUCasingLights_TrafficLightRoadSideNL_3/1

== system Demo_PreScanCarSim3D_cs/TrafficLightRoadSideNL_5 ==
  Ground_1 : Ground
  Ground_2 : Ground
  Ground_3 : Ground
  VISUCasingLights_Mux : Subsystem  Tag=MuxCasingLights
      settings: DeleteFcn=PreScanBlockDeleteFcn;
      mask Type: PreScan Mux Block:
  VISUCasingLights_TrafficLightRoadSideNL_5 : Outport  Tag=VisuCasingLightsOutport  SampleTime=20/400
  wires:
  Ground_3/1 -> VISUCasingLights_Mux/3(Green [-])
  Ground_2/1 -> VISUCasingLights_Mux/2(Orange [-])
  Ground_1/1 -> VISUCasingLights_Mux/1(Red [-])
  VISUCasingLights_Mux/1(CasingLights) -> VISUCasingLights_TrafficLightRoadSideNL_5/1

== system Demo_PreScanCarSim3D_cs/TrafficLightRoadSideNL_6 ==
  Ground_1 : Ground
  Ground_2 : Ground
  Ground_3 : Ground
  VISUCasingLights_Mux : Subsystem  Tag=MuxCasingLights
      settings: DeleteFcn=PreScanBlockDeleteFcn;
      mask Type: PreScan Mux Block:
  VISUCasingLights_TrafficLightRoadSideNL_6 : Outport  Tag=VisuCasingLightsOutport  SampleTime=20/400
  wires:
  Ground_3/1 -> VISUCasingLights_Mux/3(Green [-])
  Ground_2/1 -> VISUCasingLights_Mux/2(Orange [-])
  Ground_1/1 -> VISUCasingLights_Mux/1(Red [-])
  VISUCasingLights_Mux/1(CasingLights) -> VISUCasingLights_TrafficLightRoadSideNL_6/1

== system Demo_PreScanCarSim3D_cs/TrafficLightRoadSideNL_7 ==
  Ground_1 : Ground
  Ground_2 : Ground
  Ground_3 : Ground
  VISUCasingLights_Mux : Subsystem  Tag=MuxCasingLights
      settings: DeleteFcn=PreScanBlockDeleteFcn;
      mask Type: PreScan Mux Block:
  VISUCasingLights_TrafficLightRoadSideNL_7 : Outport  Tag=VisuCasingLightsOutport  SampleTime=20/400
  wires:
  Ground_3/1 -> VISUCasingLights_Mux/3(Green [-])
  Ground_2/1 -> VISUCasingLights_Mux/2(Orange [-])
  Ground_1/1 -> VISUCasingLights_Mux/1(Red [-])
  VISUCasingLights_Mux/1(CasingLights) -> VISUCasingLights_TrafficLightRoadSideNL_7/1

== system Demo_PreScanCarSim3D_cs/VISUCasingLights_TrafficLightRoadSideNL_1 ==
  CasingLights : Inport
  Demux4 : Demux  Outputs=3
  Saturation1 : Saturate  UpperLimit=1  LowerLimit=0
  Saturation2 : Saturate  UpperLimit=1  LowerLimit=0
  Saturation3 : Saturate  UpperLimit=1  LowerLimit=0
  conv_Green : Subsystem
  conv_Orange : Subsystem
  conv_Red : Subsystem
  visu_CasingGreen : Subsystem  mask(ToSensorWorld){PortName=visu_LightCasingGreen_0, PortIndex=948, PortWidth=16, TimeStep=20/400}
      mask prompts: PortName "Port Name [-]"; PortIndex "Index [-]"; PortWidth "Port Dimensions [-]"; TimeStep "Upload Period [s]"
      mask help: Sends signal(s) from Simulink to the Sensor World
      mask Help:
      | Sends signal(s) from Simulink to the Sensor World.
      | 
      | - Port Name [-]: specifies the name of the output terminal of the Simulink block.
      | - Index [-]: specifies the start position in the output vector sent to the Sensor World
      | - Port dimensions [-]: specifies the width (number of scalars) of the output port
      | - Upload period [s]: specifies the upload period (in seconds) of the port.
      mask Display: port_label('input', 1, PortName)
  visu_CasingOrange : Subsystem  mask(ToSensorWorld){PortName=visu_LightCasingOrange_0, PortIndex=964, PortWidth=16, TimeStep=20/400}
      mask prompts: PortName "Port Name [-]"; PortIndex "Index [-]"; PortWidth "Port Dimensions [-]"; TimeStep "Upload Period [s]"
      mask help: Sends signal(s) from Simulink to the Sensor World
      mask Help:
      | Sends signal(s) from Simulink to the Sensor World.
      | 
      | - Port Name [-]: specifies the name of the output terminal of the Simulink block.
      | - Index [-]: specifies the start position in the output vector sent to the Sensor World
      | - Port dimensions [-]: specifies the width (number of scalars) of the output port
      | - Upload period [s]: specifies the upload period (in seconds) of the port.
      mask Display: port_label('input', 1, PortName)
  visu_CasingRed : Subsystem  mask(ToSensorWorld){PortName=visu_LightCasingRed_0, PortIndex=980, PortWidth=16, TimeStep=20/400}
      mask prompts: PortName "Port Name [-]"; PortIndex "Index [-]"; PortWidth "Port Dimensions [-]"; TimeStep "Upload Period [s]"
      mask help: Sends signal(s) from Simulink to the Sensor World
      mask Help:
      | Sends signal(s) from Simulink to the Sensor World.
      | 
      | - Port Name [-]: specifies the name of the output terminal of the Simulink block.
      | - Index [-]: specifies the start position in the output vector sent to the Sensor World
      | - Port dimensions [-]: specifies the width (number of scalars) of the output port
      | - Upload period [s]: specifies the upload period (in seconds) of the port.
      mask Display: port_label('input', 1, PortName)
  wires:
  CasingLights/1 -> Demux4/1
  Demux4/3 -> Saturation3/1
  Demux4/2 -> Saturation2/1
  Demux4/1 -> Saturation1/1
  Saturation1/1 -> conv_Red/1(on_off)
  Saturation2/1 -> conv_Orange/1(on_off)
  Saturation3/1 -> conv_Green/1(on_off)
  conv_Red/1(RGBcolor) -> visu_CasingRed/1(Y)
  conv_Orange/1(RGBcolor) -> visu_CasingOrange/1(Y)
  conv_Green/1(RGBcolor) -> visu_CasingGreen/1(Y)

== system Demo_PreScanCarSim3D_cs/VISUCasingLights_TrafficLightRoadSideNL_2 ==
  CasingLights : Inport
  Demux4 : Demux  Outputs=3
  Saturation1 : Saturate  UpperLimit=1  LowerLimit=0
  Saturation2 : Saturate  UpperLimit=1  LowerLimit=0
  Saturation3 : Saturate  UpperLimit=1  LowerLimit=0
  conv_Green : Subsystem
  conv_Orange : Subsystem
  conv_Red : Subsystem
  visu_CasingGreen : Subsystem  mask(ToSensorWorld){PortName=visu_LightCasingGreen_0, PortIndex=996, PortWidth=16, TimeStep=20/400}
      mask prompts: PortName "Port Name [-]"; PortIndex "Index [-]"; PortWidth "Port Dimensions [-]"; TimeStep "Upload Period [s]"
      mask help: Sends signal(s) from Simulink to the Sensor World
      mask Help:
      | Sends signal(s) from Simulink to the Sensor World.
      | 
      | - Port Name [-]: specifies the name of the output terminal of the Simulink block.
      | - Index [-]: specifies the start position in the output vector sent to the Sensor World
      | - Port dimensions [-]: specifies the width (number of scalars) of the output port
      | - Upload period [s]: specifies the upload period (in seconds) of the port.
      mask Display: port_label('input', 1, PortName)
  visu_CasingOrange : Subsystem  mask(ToSensorWorld){PortName=visu_LightCasingOrange_0, PortIndex=1012, PortWidth=16, TimeStep=20/400}
      mask prompts: PortName "Port Name [-]"; PortIndex "Index [-]"; PortWidth "Port Dimensions [-]"; TimeStep "Upload Period [s]"
      mask help: Sends signal(s) from Simulink to the Sensor World
      mask Help:
      | Sends signal(s) from Simulink to the Sensor World.
      | 
      | - Port Name [-]: specifies the name of the output terminal of the Simulink block.
      | - Index [-]: specifies the start position in the output vector sent to the Sensor World
      | - Port dimensions [-]: specifies the width (number of scalars) of the output port
      | - Upload period [s]: specifies the upload period (in seconds) of the port.
      mask Display: port_label('input', 1, PortName)
  visu_CasingRed : Subsystem  mask(ToSensorWorld){PortName=visu_LightCasingRed_0, PortIndex=1028, PortWidth=16, TimeStep=20/400}
      mask prompts: PortName "Port Name [-]"; PortIndex "Index [-]"; PortWidth "Port Dimensions [-]"; TimeStep "Upload Period [s]"
      mask help: Sends signal(s) from Simulink to the Sensor World
      mask Help:
      | Sends signal(s) from Simulink to the Sensor World.
      | 
      | - Port Name [-]: specifies the name of the output terminal of the Simulink block.
      | - Index [-]: specifies the start position in the output vector sent to the Sensor World
      | - Port dimensions [-]: specifies the width (number of scalars) of the output port
      | - Upload period [s]: specifies the upload period (in seconds) of the port.
      mask Display: port_label('input', 1, PortName)
  wires:
  CasingLights/1 -> Demux4/1
  Demux4/3 -> Saturation3/1
  Demux4/2 -> Saturation2/1
  Demux4/1 -> Saturation1/1
  Saturation1/1 -> conv_Red/1(on_off)
  Saturation2/1 -> conv_Orange/1(on_off)
  Saturation3/1 -> conv_Green/1(on_off)
  conv_Red/1(RGBcolor) -> visu_CasingRed/1(Y)
  conv_Orange/1(RGBcolor) -> visu_CasingOrange/1(Y)
  conv_Green/1(RGBcolor) -> visu_CasingGreen/1(Y)
